simulink model "Lift_model"  (R2021a)
settings: Solver=VariableStepAuto  StartTime=0.0  StopTime=15  RelTol=1e-3
settings Model: EnablePacing=on  OrderedModelArguments=off  Creator=bunce  LastModifiedBy=matteopenlington

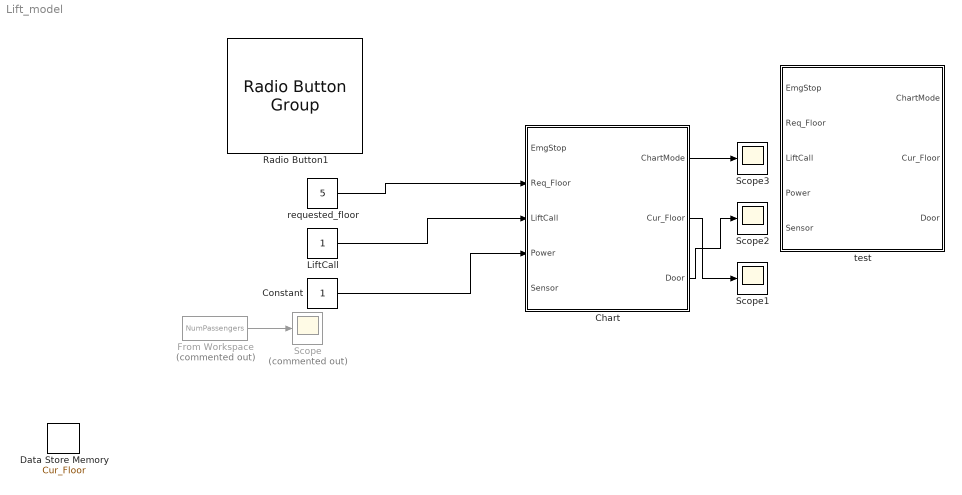
== system Lift_model ==
  Chart : Stateflow chart  TreatAsAtomicUnit=on
  Constant : Constant
  Data Store Memory : DataStoreMemory  DataStoreName=Cur_Floor  ReadBeforeWriteMsg=warning  WriteAfterWriteMsg=warning  WriteAfterReadMsg=warning  ShowAdditionalParam=off
  From Workspace : FromWorkspace  Commented=on  VariableName=NumPassengers  OutDataTypeStr=single  Interpolate=off  ZeroCross=off  OutputAfterFinalValue=Holding final value
  LiftCall : Constant
  Radio Button1 : RadioButtonGroup  SelectedLabel=5  ButtonGroupName=Group
      settings: Values={{'0', '1', '2', '3', '4', '5'}, [0 1 2 3 4 5]}
  Scope : Scope  Commented=on
  Scope1 : Scope
  Scope2 : Scope
  Scope3 : Scope
  requested_floor : Constant  Value=5
  test : Stateflow chart  TreatAsAtomicUnit=on
  wires:
  From Workspace/1 -> Scope/1
  Constant/1 -> Chart/4(Power)
  requested_floor/1 -> Chart/2(Req_Floor)
  LiftCall/1 -> Chart/3(LiftCall)
  Chart/2(Cur_Floor) -> Scope1/1
  Chart/1(ChartMode) -> Scope3/1
  Chart/3(Door) -> Scope2/1

== stateflow chart Lift_model/Chart ==
  state Initial
    entry:
    Cur_Floor = 0;
  note: This is for:
      | - lift is at floor 0.
      | - user calls lift from floor 0
      | - lift requested to floor 2
  note: The lift will always be on. The individual components may not. But the actual system will have to be. Otherwise the signals won't be read to let the lift know what to do.
  state Off [commented out]
  state Idle_doors
    entry:
    exit:
    state DoorOpen
      entry:
      Door = 1;
    state DoorClose
      exit:
      Door = 0;
    (default) -> Idle_doors.DoorOpen
    Idle_doors.DoorClose -> Idle_doors.DoorOpen [order 1] : [Door == 0 || Sensor == 1]
    Idle_doors.DoorOpen -> Idle_doors.DoorClose : [Door == 1]
    Idle_doors.DoorClose -> Idle_doors [order 2] : [Door == 0 && Sensor == 0]
  state Idle_waiting
  state On [commented out]
    exit:
    Motor == 0;
    state Idle [commented out]
      state DoorOpen [commented out]
      state DoorClose [commented out]
      (default) -> On.Idle.DoorOpen [commented out]
      On.Idle.DoorClose -> On.Idle.DoorOpen [commented out] : [Door == 0 || Sensor == 1]
      On.Idle.DoorOpen -> On.Idle.DoorClose [commented out] : [Door == 1]
    state MovingUp [commented out]
      entry:
      Motor == 1;
      exit:
      Motor == 0;
    state MovingDown [commented out]
      entry:
      Motor == -1;
      exit:
      Motor == 0;
    (default) -> Idle [commented out]
    Idle -> On.MovingUp [commented out]
    On.MovingUp -> Idle [commented out]
    Idle -> On.MovingDown [commented out]
    On.MovingDown -> Idle [commented out]
  state MovingUp
    entry:
    %Motor == 1;
    exit:
    %Motor == 0;
  state MovingDown
    entry:
    %Motor == -1;
    exit:
    %Motor == 0;
  state Error [commented out]
    entry:
    EmgStop == 1;
    Motor == 0;
  (default) -> Initial
  Initial -> (junction 55)
  (junction 55) -> Idle_waiting [order 2] : [LiftCall ~= 1]
  (default) -> Off [commented out]
  (junction 55) -> Idle_doors [order 1] : [LiftCall == 1]
  Off -> On [commented out] : [Power == 1 && Error == 0]
  Idle_doors -> MovingUp [order 1] : [Req_Floor > Cur_Floor]
  MovingUp -> Idle_doors : after(2,sec){Cur_Floor = Cur_Floor + 1}
  Idle_doors -> MovingDown [order 2] : [Req_Floor > Cur_Floor]
  MovingDown -> Idle_doors : after(2,sec){Cur_Floor = Cur_Floor - 1}
  On -> Off [commented out] : [Power == 0]
  Error -> Off [commented out] : after(30,sec)
  On -> Error [commented out] : [Error == 1]
  data: ChartMode output Enum: ChartModeType; EmgStop input; Req_Floor input; LiftCall input; Power input; Sensor input; Cur_Floor output double; Door output

== stateflow chart Lift_model/test ==
  state Initial
    entry:
    Cur_Floor = 0;
  note: This is for:
      | - lift is at floor 0.
      | - user calls lift from floor 0
      | - lift requested to floor 2
  note: The lift will always be on. The individual components may not. But the actual system will have to be. Otherwise the signals won't be read to let the lift know what to do.
  state Off [commented out]
  state Idle_doors
    entry:
    exit:
    state DoorOpen
      entry:
      Door = 1;
    state DoorClose
      exit:
      Door = 0;
    (default) -> Idle_doors.DoorOpen
    Idle_doors.DoorClose -> Idle_doors.DoorOpen [order 1] : [Door == 0 || Sensor == 1]
    Idle_doors.DoorOpen -> Idle_doors.DoorClose : [Door == 1]
    Idle_doors.DoorClose -> Idle_doors [order 2] : [Door == 0 && Sensor == 0]
  state Idle_waiting
  state On [commented out]
    exit:
    Motor == 0;
    state Idle [commented out]
      state DoorOpen [commented out]
      state DoorClose [commented out]
      (default) -> On.Idle.DoorOpen [commented out]
      On.Idle.DoorClose -> On.Idle.DoorOpen [commented out] : [Door == 0 || Sensor == 1]
      On.Idle.DoorOpen -> On.Idle.DoorClose [commented out] : [Door == 1]
    state MovingUp [commented out]
      entry:
      Motor == 1;
      exit:
      Motor == 0;
    state MovingDown [commented out]
      entry:
      Motor == -1;
      exit:
      Motor == 0;
    (default) -> Idle [commented out]
    Idle -> On.MovingUp [commented out]
    On.MovingUp -> Idle [commented out]
    Idle -> On.MovingDown [commented out]
    On.MovingDown -> Idle [commented out]
  state MovingUp
    entry:
    %Motor == 1;
    exit:
    %Motor == 0;
  state MovingDown
    entry:
    %Motor == -1;
    exit:
    %Motor == 0;
  state Error [commented out]
    entry:
    EmgStop == 1;
    Motor == 0;
  (default) -> Initial
  Initial -> (junction 55)
  (junction 55) -> Idle_waiting [order 2] : [LiftCall ~= 1]
  (default) -> Off [commented out]
  (junction 55) -> Idle_doors [order 1] : [LiftCall == 1]
  Off -> On [commented out] : [Power == 1 && Error == 0]
  Idle_doors -> MovingUp [order 1] : [Req_Floor > Cur_Floor]
  MovingUp -> Idle_doors : after(2,sec){Cur_Floor = Cur_Floor + 1}
  Idle_doors -> MovingDown [order 2] : [Req_Floor > Cur_Floor]
  MovingDown -> Idle_doors : after(2,sec){Cur_Floor = Cur_Floor - 1}
  On -> Off [commented out] : [Power == 0]
  Error -> Off [commented out] : after(30,sec)
  On -> Error [commented out] : [Error == 1]
  data: ChartMode output Enum: ChartModeType; EmgStop input; Req_Floor input; LiftCall input; Power input; Sensor input; Cur_Floor output double; Door output
